simulink model "closed_loop_motor"  (R2021a)
settings: Solver=VariableStepAuto  StartTime=0.0  StopTime=30  RelTol=1e-3
values from neighbouring files (symbols this model uses):
  airDensity = 1.225    [mobile_robot_data.mat]
  desiredSpeed_kmh = 5    [mobile_robot_data.mat]
  dragCoefficient = 0.1    [mobile_robot_data.mat]
  efficiency = 0.4    [mobile_robot_data.mat]
  frontalArea = 0.1    [mobile_robot_data.mat]
  gearRatio = 2.4154589372    [mobile_robot_data.mat]
  inclineForce = 0    [mobile_robot_data.mat]
  nominalVoltage = 18    [mobile_robot_data.mat]
  numberOfWheels = 4    [mobile_robot_data.mat]
  robotWeight = 30    [mobile_robot_data.mat]
  rollingResistanceForce = 8.829    [mobile_robot_data.mat]
  speedConstant = 255    [mobile_robot_data.mat]
  stallCurrent = 76.3    [mobile_robot_data.mat]
  static_coeff = 0.7    [mobile_robot_data.mat]
  terminalInductance = 0.169    [mobile_robot_data.mat]
  terminalResistance = 0.236    [mobile_robot_data.mat]
  torqueConstant = 37.5    [mobile_robot_data.mat]
  wheelRadius = 0.1    [mobile_robot_data.mat]
libraries: simulink x1, dspstat3 x1, pid_lib x1
settings Model: Creator=Muhammed  LastModifiedBy=Muhammed

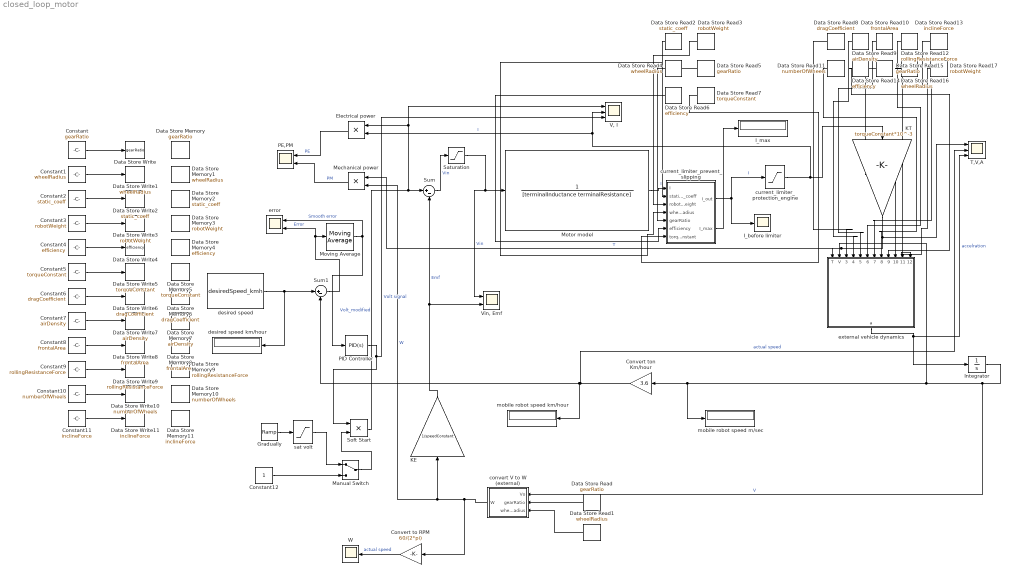
== system closed_loop_motor ==
  Constant : Constant  Value=gearRatio
  Constant1 : Constant  Value=wheelRadius
  Constant10 : Constant  Value=numberOfWheels
  Constant11 : Constant  Value=inclineForce
  Constant12 : Constant
  Constant2 : Constant  Value=static_coeff
  Constant3 : Constant  Value=robotWeight
  Constant4 : Constant  Value=efficiency
  Constant5 : Constant  Value=torqueConstant
  Constant6 : Constant  Value=dragCoefficient
  Constant7 : Constant  Value=airDensity
  Constant8 : Constant  Value=frontalArea
  Constant9 : Constant  Value=rollingResistanceForce
  Convert to RPM : Gain  Gain=60/(2*pi)
  Convert ton Km/hour : Gain  Gain=3.6
  Data Store Memory : DataStoreMemory  DataStoreName=gearRatio  ReadBeforeWriteMsg=warning  WriteAfterWriteMsg=warning  WriteAfterReadMsg=warning  ShowAdditionalParam=off
  Data Store Memory1 : DataStoreMemory  DataStoreName=wheelRadius  ReadBeforeWriteMsg=warning  WriteAfterWriteMsg=warning  WriteAfterReadMsg=warning  ShowAdditionalParam=off
  Data Store Memory10 : DataStoreMemory  DataStoreName=numberOfWheels  ReadBeforeWriteMsg=warning  WriteAfterWriteMsg=warning  WriteAfterReadMsg=warning  ShowAdditionalParam=off
  Data Store Memory11 : DataStoreMemory  DataStoreName=inclineForce  ReadBeforeWriteMsg=warning  WriteAfterWriteMsg=warning  WriteAfterReadMsg=warning  ShowAdditionalParam=off
  Data Store Memory2 : DataStoreMemory  DataStoreName=static_coeff  ReadBeforeWriteMsg=warning  WriteAfterWriteMsg=warning  WriteAfterReadMsg=warning  ShowAdditionalParam=off
  Data Store Memory3 : DataStoreMemory  DataStoreName=robotWeight  ReadBeforeWriteMsg=warning  WriteAfterWriteMsg=warning  WriteAfterReadMsg=warning  ShowAdditionalParam=off
  Data Store Memory4 : DataStoreMemory  DataStoreName=efficiency  ReadBeforeWriteMsg=warning  WriteAfterWriteMsg=warning  WriteAfterReadMsg=warning  ShowAdditionalParam=off
  Data Store Memory5 : DataStoreMemory  DataStoreName=torqueConstant  ReadBeforeWriteMsg=warning  WriteAfterWriteMsg=warning  WriteAfterReadMsg=warning  ShowAdditionalParam=off
  Data Store Memory6 : DataStoreMemory  DataStoreName=dragCoefficient  ReadBeforeWriteMsg=warning  WriteAfterWriteMsg=warning  WriteAfterReadMsg=warning  ShowAdditionalParam=off
  Data Store Memory7 : DataStoreMemory  DataStoreName=airDensity  ReadBeforeWriteMsg=warning  WriteAfterWriteMsg=warning  WriteAfterReadMsg=warning  ShowAdditionalParam=off
  Data Store Memory8 : DataStoreMemory  DataStoreName=frontalArea  ReadBeforeWriteMsg=warning  WriteAfterWriteMsg=warning  WriteAfterReadMsg=warning  ShowAdditionalParam=off
  Data Store Memory9 : DataStoreMemory  DataStoreName=rollingResistanceForce  ReadBeforeWriteMsg=warning  WriteAfterWriteMsg=warning  WriteAfterReadMsg=warning  ShowAdditionalParam=off
  Data Store Read : DataStoreRead  DataStoreName=gearRatio  IndexOptions=Index vector (dialog)  Indices=1  OutputSizes=1
  Data Store Read1 : DataStoreRead  DataStoreName=wheelRadius  IndexOptions=Index vector (dialog)  Indices=1  OutputSizes=1
  Data Store Read10 : DataStoreRead  DataStoreName=frontalArea  IndexOptions=Index vector (dialog)  Indices=1  OutputSizes=1
  Data Store Read11 : DataStoreRead  DataStoreName=numberOfWheels  IndexOptions=Index vector (dialog)  Indices=1  OutputSizes=1
  Data Store Read12 : DataStoreRead  DataStoreName=rollingResistanceForce  IndexOptions=Index vector (dialog)  Indices=1  OutputSizes=1
  Data Store Read13 : DataStoreRead  DataStoreName=inclineForce  IndexOptions=Index vector (dialog)  Indices=1  OutputSizes=1
  Data Store Read14 : DataStoreRead  DataStoreName=efficiency  IndexOptions=Index vector (dialog)  Indices=1  OutputSizes=1
  Data Store Read15 : DataStoreRead  DataStoreName=gearRatio  IndexOptions=Index vector (dialog)  Indices=1  OutputSizes=1
  Data Store Read16 : DataStoreRead  DataStoreName=wheelRadius  IndexOptions=Index vector (dialog)  Indices=1  OutputSizes=1
  Data Store Read17 : DataStoreRead  DataStoreName=robotWeight  IndexOptions=Index vector (dialog)  Indices=1  OutputSizes=1
  Data Store Read2 : DataStoreRead  DataStoreName=static_coeff  IndexOptions=Index vector (dialog)  Indices=1  OutputSizes=1
  Data Store Read3 : DataStoreRead  DataStoreName=robotWeight  IndexOptions=Index vector (dialog)  Indices=1  OutputSizes=1
  Data Store Read4 : DataStoreRead  DataStoreName=wheelRadius  IndexOptions=Index vector (dialog)  Indices=1  OutputSizes=1
  Data Store Read5 : DataStoreRead  DataStoreName=gearRatio  IndexOptions=Index vector (dialog)  Indices=1  OutputSizes=1
  Data Store Read6 : DataStoreRead  DataStoreName=efficiency  IndexOptions=Index vector (dialog)  Indices=1  OutputSizes=1
  Data Store Read7 : DataStoreRead  DataStoreName=torqueConstant  IndexOptions=Index vector (dialog)  Indices=1  OutputSizes=1
  Data Store Read8 : DataStoreRead  DataStoreName=dragCoefficient  IndexOptions=Index vector (dialog)  Indices=1  OutputSizes=1
  Data Store Read9 : DataStoreRead  DataStoreName=airDensity  IndexOptions=Index vector (dialog)  Indices=1  OutputSizes=1
  Data Store Write : DataStoreWrite  DataStoreName=gearRatio  IndexOptions=Index vector (dialog)  Indices=1  OutputSizes=1
  Data Store Write1 : DataStoreWrite  DataStoreName=wheelRadius  IndexOptions=Index vector (dialog)  Indices=1  OutputSizes=1
  Data Store Write10 : DataStoreWrite  DataStoreName=numberOfWheels  IndexOptions=Index vector (dialog)  Indices=1  OutputSizes=1
  Data Store Write11 : DataStoreWrite  DataStoreName=inclineForce  IndexOptions=Index vector (dialog)  Indices=1  OutputSizes=1
  Data Store Write2 : DataStoreWrite  DataStoreName=static_coeff  IndexOptions=Index vector (dialog)  Indices=1  OutputSizes=1
  Data Store Write3 : DataStoreWrite  DataStoreName=robotWeight  IndexOptions=Index vector (dialog)  Indices=1  OutputSizes=1
  Data Store Write4 : DataStoreWrite  DataStoreName=efficiency  IndexOptions=Index vector (dialog)  Indices=1  OutputSizes=1
  Data Store Write5 : DataStoreWrite  DataStoreName=torqueConstant  IndexOptions=Index vector (dialog)  Indices=1  OutputSizes=1
  Data Store Write6 : DataStoreWrite  DataStoreName=dragCoefficient  IndexOptions=Index vector (dialog)  Indices=1  OutputSizes=1
  Data Store Write7 : DataStoreWrite  DataStoreName=airDensity  IndexOptions=Index vector (dialog)  Indices=1  OutputSizes=1
  Data Store Write8 : DataStoreWrite  DataStoreName=frontalArea  IndexOptions=Index vector (dialog)  Indices=1  OutputSizes=1
  Data Store Write9 : DataStoreWrite  DataStoreName=rollingResistanceForce  IndexOptions=Index vector (dialog)  Indices=1  OutputSizes=1
  Electrical power : Product
  Gradually : simulink/Sources/Ramp  slope=2  start=0  InitialOutput=0
  I_before limiter : Scope
  I_max : Display
  Integrator : Integrator
  KE : Gain  Gain=1/speedConstant
  KT : Gain  Gain=torqueConstant*10^-3
  Manual Switch : ManualSwitch
  Mechanical power : Product
  Motor model : TransferFcn  Denominator=[terminalInductance terminalResistance]
  Moving Average : dspstat3/Moving Average  Method=Sliding window  ForgettingFactorPort=off  SpecifyWindowLength=on  WindowLength=5  ForgettingFactor=0.9  SimulateUsing=Code generation
  PE,PM : Scope  NumInputPorts=2
  PID Controller : pid_lib/PID Controller  Controller=PID  Form=Parallel  TimeDomain=Continuous-time  UseExternalTs=off  SampleTime=-1  IntegratorMethod=Forward Euler  FilterMethod=Forward Euler  ControllerParametersSource=internal  P=3  I=0.168  D=2  UseFilter=on  N=15  TunerSelectOption=Frequency Response Based  InitialConditionSource=internal  InitialConditionForIntegrator=0  InitialConditionForFilter=0  DifferentiatorICPrevScaledInput=0  ExternalReset=none  TrackingMode=off  Kt=1  LimitOutput=on  SatLimitsSource=internal  UpperSaturationLimit=nominalVoltage  LowerSaturationLimit=0  LinearizeAsGain=on  AntiWindupMode=none  Kb=1  POutMin=[]  POutMax=[]  IOutMin=[]  IOutMax=[]  DOutMin=[]  DOutMax=[]  NOutMin=[]  NOutMax=[]  SumOutMin=[]  SumOutMax=[]  SaturationOutMin=[]  SaturationOutMax=[]  PParamMin=[]  PParamMax=[]  IParamMin=[]  IParamMax=[]  DParamMin=[]  DParamMax=[]  NParamMin=[]  NParamMax=[]  KbParamMin=[]  KbParamMax=[]  KtParamMin=[]  KtParamMax=[]  KbOutMin=[]  KbOutMax=[]  KtOutMin=[]  KtOutMax=[]  IntegratorOutMin=[]  IntegratorOutMax=[]  FilterOutMin=[]  FilterOutMax=[]  SumI1OutMin=[]  SumI1OutMax=[]  SumI2OutMin=[]  SumI2OutMax=[]  SumI3OutMin=[]  SumI3OutMax=[]  SumI4OutMin=[]  SumI4OutMax=[]  SumDOutMin=[]  SumDOutMax=[]  DifferentiatorOutMin=[]  DifferentiatorOutMax=[]  FilterDiffOutCoefMin=[]  FilterDiffOutCoefMax=[]  ReciprocalOutMin=[]  ReciprocalOutMax=[]  SumDenOutMin=[]  SumDenOutMax=[]  SumNumOutMin=[]  SumNumOutMax=[]  DivideOutMin=[]  DivideOutMax=[]  UdiffTsProdOutMin=[]  UdiffTsProdOutMax=[]  NTsProdOutMin=[]  NTsProdOutMax=[]  UintegralTsProdOutMin=[]  UintegralTsProdOutMax=[]  UngainTsProdOutMin=[]  UngainTsProdOutMax=[]  IntegratorContinuousStateAttributes=''  IntegratorStateMustResolveToSignalObject=off  IntegratorRTWStateStorageClass=Auto  FilterContinuousStateAttributes=''  FilterStateMustResolveToSignalObject=off  FilterRTWStateStorageClass=Auto  ParallelPVariant=InternalParameters  IdealPVariant=Disabled  IVariant=InternalParameters  DVariant=InternalParameters  IntegratorVariant=Continuous  SatVariant=Enabled  AWVariant=Passthrough  PCopyVariant=Disabled  TRVariant=Disabled  FdbkBlocksVariant=Forward  IdealPFdbkVariant=Disabled  SatFdbkVariant=Disabled  DerivativeFilterVariant=ContFilter  NVariant=InternalParameters  NCopyVariant=Disabled  FilterICVariant=InternalICsFilter  IntegratorICVariant=InternalICs  ExternalResetVariant=Disabled  TRSumVariant=Passthrough  SumFdbkVariant=Disabled  SumVariant=Sum_PID  TsampFilterVariant=InternalTs  TsampNgainVariant=Passthrough  TsampIntegralVariant=Passthrough  ExternalSaturationOutDataTypeStr=Inherit: Same as second input
  Saturation : Saturate  UpperLimit=nominalVoltage  LowerLimit=0
  Soft Start : Product
  Sum : Sum  Inputs=|+-
  Sum1 : Sum  Inputs=|+-
  T,V,A : Scope  NumInputPorts=3
  "V, I" : Scope  NumInputPorts=3
  "Vin, Emf" : Scope  NumInputPorts=2
  W : Scope
  convert V to W (external) : MATLAB Function  TreatAsAtomicUnit=on
  current_limiter_prevent_slipping : MATLAB Function  TreatAsAtomicUnit=on
  current_limiter_protection_engine : Saturate  UpperLimit=0.7 * stallCurrent  LowerLimit=0
  desired speed : Constant  Value=desiredSpeed_kmh
  desired speed km/hour : Display
  error : Scope  NumInputPorts=2
  external vehicle dynamics : MATLAB Function  TreatAsAtomicUnit=on
  mobile robot speed km/hour : Display
  mobile robot speed m/sec : Display
  sat volt : Saturate  UpperLimit=1  LowerLimit=0
  wires:
  Convert to RPM/1 -> W/1  "actual speed"
  Saturation/1 -> "Vin, Emf"/1, Motor model/1  "Vin"
  Data Store Read16/1 -> external vehicle dynamics/11(wheelRadius)
  Constant10/1 -> Data Store Write10/1
  Constant2/1 -> Data Store Write2/1
  Data Store Read11/1 -> external vehicle dynamics/8(numberOfWheels)
  Constant6/1 -> Data Store Write6/1
  Data Store Read10/1 -> external vehicle dynamics/5(frontalArea)
  Data Store Read3/1 -> current_limiter_prevent_slipping/3(robotWeight)
  Constant8/1 -> Data Store Write8/1
  Constant11/1 -> Data Store Write11/1
  Data Store Read5/1 -> current_limiter_prevent_slipping/5(gearRatio)
  external vehicle dynamics/1(a) -> T,V,A/3, Integrator/1  "accelration"
  Constant7/1 -> Data Store Write7/1
  Data Store Read14/1 -> external vehicle dynamics/9(efficiency)
  Data Store Read15/1 -> external vehicle dynamics/10(gearRatio)
  current_limiter_protection_engine/1 -> "V, I"/2, Electrical power/2, KT/1  "I"
  Data Store Read4/1 -> current_limiter_prevent_slipping/4(wheelRadius)
  KE/1 -> "Vin, Emf"/2, Sum/2  "Emf"
  Data Store Read17/1 -> external vehicle dynamics/12(robotWeight)
  Constant/1 -> Data Store Write/1
  Constant5/1 -> Data Store Write5/1
  Mechanical power/1 -> PE,PM/2  "PM"
  Data Store Read7/1 -> current_limiter_prevent_slipping/7(torqueConstant)
  Data Store Read8/1 -> external vehicle dynamics/3(dragCoefficient)
  Data Store Read12/1 -> external vehicle dynamics/6(rollingResistanceForce)
  Electrical power/1 -> PE,PM/1  "PE"
  Sum/1 -> Saturation/1  "Vin"
  Constant3/1 -> Data Store Write3/1
  current_limiter_prevent_slipping/2(I_max) -> I_max/1
  desired speed/1 -> desired speed km/hour/1, Sum1/1
  Data Store Read1/1 -> convert V to W (external)/3(wheelRadius)
  current_limiter_prevent_slipping/1(I_out) -> current_limiter_protection_engine/1, I_before limiter/1  "I"
  Motor model/1 -> current_limiter_prevent_slipping/1(I)  "I"
  Data Store Read13/1 -> external vehicle dynamics/7(inclineForce)
  Integrator/1 -> convert V to W (external)/1(Vo), external vehicle dynamics/2(V), mobile robot speed m/sec/1, Convert ton Km/hour/1  "V"
  Convert ton Km/hour/1 -> T,V,A/2, Sum1/2, mobile robot speed km/hour/1  "actual speed"
  KT/1 -> Mechanical power/1, external vehicle dynamics/1(T), T,V,A/1  "T"
  convert V to W (external)/1(W) -> Convert to RPM/1, Mechanical power/2, KE/1  "W"
  Constant4/1 -> Data Store Write4/1
  Data Store Read9/1 -> external vehicle dynamics/4(airDensity)
  Data Store Read6/1 -> current_limiter_prevent_slipping/6(efficiency)
  Data Store Read2/1 -> current_limiter_prevent_slipping/2(static_coeff)
  Data Store Read/1 -> convert V to W (external)/2(gearRatio)
  Constant9/1 -> Data Store Write9/1
  Constant1/1 -> Data Store Write1/1
  Gradually/1 -> sat volt/1
  sat volt/1 -> Manual Switch/1
  Constant12/1 -> Manual Switch/2
  Manual Switch/1 -> Soft Start/2
  PID Controller/1 -> Soft Start/1, "V, I"/3  "Volt signal"
  Soft Start/1 -> "V, I"/1, Electrical power/1, Sum/1  "Volt_modified"
  Sum1/1 -> error/2, Moving Average/1  "Error"
  Moving Average/1 -> PID Controller/1, error/1  "Smooth error"

== matlab function closed_loop_motor/current_limiter_prevent_slipping ==
  data: I input; I_out output; I_max output; static_coeff input; robotWeight input; wheelRadius input; gearRatio input; efficiency input; torqueConstant input
function [I_out, I_max] = current_limiter(I, static_coeff, robotWeight, wheelRadius, gearRatio, efficiency, torqueConstant)
    

    
    F_max = static_coeff * robotWeight * 9.81;
    % Calculate maximum torque from maximum static force
    T_max = F_max * wheelRadius / (gearRatio * efficiency);
    
    % Calculate maximum current from maximum torque
    I_max = T_max / (torqueConstant * 10^-3);
    
    % Saturate input current with calculated maximum current
    I_out = min(I, I_max);
end

== matlab function closed_loop_motor/external vehicle dynamics ==
  data: T input; a output; V input; dragCoefficient input; airDensity input; frontalArea input; rollingResistanceForce input; inclineForce input; numberOfWheels input; efficiency input; gearRatio input; wheelRadius input; robotWeight input
function a = fcn(T, V, dragCoefficient, airDensity, frontalArea, rollingResistanceForce, inclineForce, numberOfWheels, efficiency, gearRatio, wheelRadius, robotWeight)



c =  0.5 * dragCoefficient * airDensity * frontalArea;
Fd = c * V ^2;

Fr = rollingResistanceForce;
Fi = inclineForce;

F_traction = numberOfWheels * (efficiency * gearRatio * T ) / wheelRadius; 
a  = (F_traction - Fr - Fd - Fi) / robotWeight;

== matlab function closed_loop_motor/convert V to W (external) ==
  data: Vo input; W output; gearRatio input; wheelRadius input
function W = fcn(Vo, gearRatio, wheelRadius)


W  = (Vo * gearRatio) / wheelRadius ;
